simulink model "MAY31v1"  (R2023a)
settings: Solver=ode23t  StartTime=0.0  StopTime=1.6  RelTol=1e-3  AbsTol=1e-4  EnableMultiTasking=on
InitFcn:
  | Scan_Script_v8
StopFcn:
  | graphB
model workspace (MATLAB code in the model file):
  | screw_lead = 25e-3;   % m/rev
values from neighbouring files (symbols this model uses):
  mx = 1.557096    [Parameters.m]
  my = 0.574990    (= 0.57499)    [Parameters.m]
  mz = 1.557196    [Parameters.m]
  R_D = 1e-2    (= 0.01)    [Parameters.m]
  R_I = 1.2*1e-6    (= 1.2e-06)    [Parameters.m]
  Step_Rate = 200    [Parameters.m]
undefined symbols (not defined in the file or in its folder): X, xz, Y, y, Z
libraries: fl_lib x72, nesl_utility x58, sm_lib x41, fl_ps_legacy_lib x24, ee_lib x6, simulink x3, eeStairGenerator x3
(part 3 of 3)

== system MAY31v1/Stepper Motor with Control Y/Controller/Speed ==
  note: Step rate and direction algorithm implemented on a microprocessor or dedicated discrete chip
  Ref : Inport
  ERef : fl_lib/Electrical/Electrical Elements/Electrical Reference
  Step Rate and Direction : Subsystem
  Voltage-Controlled Pulse Generator : Subsystem
  PWM : PMIOPort  Side=Right
  0v : PMIOPort  Port=2  Side=Right
  REV : PMIOPort  Port=3  Side=Right
  wires:
  Ref/1 -> Step Rate and Direction/1(Reference)
  connections:
  PWM/RConn1 -- Voltage-Controlled Pulse Generator/RConn1
  Voltage-Controlled Pulse Generator/RConn2 -- 0v/RConn1 -- ERef/LConn1
  Step Rate and Direction/RConn1 -- REV/RConn1
  Step Rate and Direction/RConn2 -- Voltage-Controlled Pulse Generator/LConn1

== system MAY31v1/Stepper Motor with Control Z/Controller/Position ==
  Ref : Inport
  Algorithm and Pulse Generation : Subsystem
  ERef : fl_lib/Electrical/Electrical Elements/Electrical Reference
  PWM : PMIOPort  Side=Right
  0v : PMIOPort  Port=2  Side=Right
  REV : PMIOPort  Port=3  Side=Right
  wires:
  Ref/1 -> Algorithm and Pulse Generation/1(Reference)
  connections:
  Algorithm and Pulse Generation/RConn2 -- PWM/RConn1
  Algorithm and Pulse Generation/RConn1 -- REV/RConn1
  ERef/LConn1 -- 0v/RConn1

== system MAY31v1/Stepper Motor with Control Z/Controller/Speed ==
  note: Step rate and direction algorithm implemented on a microprocessor or dedicated discrete chip
  Ref : Inport
  ERef : fl_lib/Electrical/Electrical Elements/Electrical Reference
  Step Rate and Direction : Subsystem
  Voltage-Controlled Pulse Generator : Subsystem
  PWM : PMIOPort  Side=Right
  0v : PMIOPort  Port=2  Side=Right
  REV : PMIOPort  Port=3  Side=Right
  wires:
  Ref/1 -> Step Rate and Direction/1(Reference)
  connections:
  PWM/RConn1 -- Voltage-Controlled Pulse Generator/RConn1
  Voltage-Controlled Pulse Generator/RConn2 -- 0v/RConn1 -- ERef/LConn1
  Step Rate and Direction/RConn1 -- REV/RConn1
  Step Rate and Direction/RConn2 -- Voltage-Controlled Pulse Generator/LConn1

== system MAY31v1/X axis Lead Screw/Lead Screw Friction/Lag Filter ==
  In : Inport
  Gain : Gain  Gain=1/b
  Integrator : Integrator  InitialCondition=x_initial
  Sum : Sum  Inputs=|+-  InputSameDT=on  SaturateOnIntegerOverflow=on  OutDataTypeStr=Inherit: Same as first input
  Out : Outport  VectorParamsAs1DForOutWhenUnconnected=off
  wires:
  Sum/1 -> Integrator/1
  In/1 -> Sum/1
  Integrator/1 -> Gain/1
  Gain/1 -> Sum/2, Out/1

== system MAY31v1/X axis Lead Screw/Lead Screw Friction/Stick-Slip Friction  ==
  Fn : Inport
  v : Inport  Port=2
  Coefficient of Friction vs Velocity : Lookup_n-D  NumberOfTableDimensions=1  BreakpointsForDimension1=[-3 -1.5 -1 1 1.5 3]*vth  Table="[-muk -muk -mus mus  muk muk]"  InternalRulePriority=Speed
  Gain2 : Gain  Multiplication=Matrix(K*u)  SaturateOnIntegerOverflow=on  OutDataTypeStr=Inherit: Same as input  ParamDataTypeStr=Inherit: Same as input
  Product : Product  RndMeth=Zero
  Ff : Outport  VectorParamsAs1DForOutWhenUnconnected=off
  wires:
  Fn/1 -> Product/2  "Normal_Force"
  Coefficient of Friction vs Velocity/1 -> Product/1
  v/1 -> Coefficient of Friction vs Velocity/1  "Velocity"
  Product/1 -> Gain2/1
  Gain2/1 -> Ff/1  "Friction_Force"

== system MAY31v1/Y Axis Lead Screw/Lead Screw Friction2/Lag Filter ==
  In : Inport
  Gain : Gain  Gain=1/b
  Integrator : Integrator  InitialCondition=x_initial
  Sum : Sum  Inputs=|+-  InputSameDT=on  SaturateOnIntegerOverflow=on  OutDataTypeStr=Inherit: Same as first input
  Out : Outport  VectorParamsAs1DForOutWhenUnconnected=off
  wires:
  Sum/1 -> Integrator/1
  In/1 -> Sum/1
  Integrator/1 -> Gain/1
  Gain/1 -> Sum/2, Out/1

== system MAY31v1/Y Axis Lead Screw/Lead Screw Friction2/Stick-Slip Friction  ==
  Fn : Inport
  v : Inport  Port=2
  Coefficient of Friction vs Velocity : Lookup_n-D  NumberOfTableDimensions=1  BreakpointsForDimension1=[-3 -1.5 -1 1 1.5 3]*vth  Table="[-muk -muk -mus mus  muk muk]"  InternalRulePriority=Speed
  Gain2 : Gain  Multiplication=Matrix(K*u)  SaturateOnIntegerOverflow=on  OutDataTypeStr=Inherit: Same as input  ParamDataTypeStr=Inherit: Same as input
  Product : Product  RndMeth=Zero
  Ff : Outport  VectorParamsAs1DForOutWhenUnconnected=off
  wires:
  Fn/1 -> Product/2  "Normal_Force"
  Coefficient of Friction vs Velocity/1 -> Product/1
  v/1 -> Coefficient of Friction vs Velocity/1  "Velocity"
  Product/1 -> Gain2/1
  Gain2/1 -> Ff/1  "Friction_Force"

== system MAY31v1/Z axis Lead Screw/Lead Screw Friction1/Lag Filter ==
  In : Inport
  Gain : Gain  Gain=1/b
  Integrator : Integrator  InitialCondition=x_initial
  Sum : Sum  Inputs=|+-  InputSameDT=on  SaturateOnIntegerOverflow=on  OutDataTypeStr=Inherit: Same as first input
  Out : Outport  VectorParamsAs1DForOutWhenUnconnected=off
  wires:
  Sum/1 -> Integrator/1
  In/1 -> Sum/1
  Integrator/1 -> Gain/1
  Gain/1 -> Sum/2, Out/1

== system MAY31v1/Z axis Lead Screw/Lead Screw Friction1/Stick-Slip Friction  ==
  Fn : Inport
  v : Inport  Port=2
  Coefficient of Friction vs Velocity : Lookup_n-D  NumberOfTableDimensions=1  BreakpointsForDimension1=[-3 -1.5 -1 1 1.5 3]*vth  Table="[-muk -muk -mus mus  muk muk]"  InternalRulePriority=Speed
  Gain2 : Gain  Multiplication=Matrix(K*u)  SaturateOnIntegerOverflow=on  OutDataTypeStr=Inherit: Same as input  ParamDataTypeStr=Inherit: Same as input
  Product : Product  RndMeth=Zero
  Ff : Outport  VectorParamsAs1DForOutWhenUnconnected=off
  wires:
  Fn/1 -> Product/2  "Normal_Force"
  Coefficient of Friction vs Velocity/1 -> Product/1
  v/1 -> Coefficient of Friction vs Velocity/1  "Velocity"
  Product/1 -> Gain2/1
  Gain2/1 -> Ff/1  "Friction_Force"

== system MAY31v1/Stepper Motor with Control X/Controller/Position/Algorithm and Pulse Generation ==
  note: The reference input defines the required angular position in terms of
      | the number steps. For this stepper, the step size is 1.8 degrees. Hence
      | a demand of 10 steps results in an angle change of 18 degrees.
      | The step rate is set by the Pulse Generator's Pulse rate mask parameter.
  note: Position Controller
  Reference : Inport
  IC Analog Output REV : Subsystem
  IC Analog Output Vref : Subsystem
  Logic2Volts1 : Gain  Gain=5
  Logic2Volts2 : Gain  Gain=5
  Pulse Generator : Subsystem  mask{f=Step_Rate}
      mask prompts: f "Pulse rate"
  Rate Transition : RateTransition  Deterministic=off
  REV : PMIOPort  Side=Right
  Vref : PMIOPort  Port=2  Side=Right
  wires:
  Logic2Volts1/1 -> IC Analog Output Vref/1(SL)
  Pulse Generator/1(Pulse train) -> Logic2Volts1/1
  Reference/1 -> Rate Transition/1
  Logic2Volts2/1 -> IC Analog Output REV/1(SL)
  Pulse Generator/2(Pulse direction) -> Logic2Volts2/1
  Rate Transition/1 -> Pulse Generator/1(Pulse  demand)
  connections:
  Vref/RConn1 -- IC Analog Output Vref/RConn1
  REV/RConn1 -- IC Analog Output REV/RConn1

== system MAY31v1/Stepper Motor with Control X/Controller/Speed/Step Rate and Direction ==
  note: The speed controller turns the reference input into an absolute voltage demand for the
      | voltage-controlled pulse generator and sets the reverse flag signal to +5 volts when the
      | speed demand is negative.
  Reference : Inport
  Abs : Abs  SaturateOnIntegerOverflow=off
  Compare To Constant : simulink/Logic and Bit Operations/Compare To Constant  relop=<  const=0  OutDataTypeStr=uint8  ZeroCross=off
  Data Type Conversion : DataTypeConversion  SaturateOnIntegerOverflow=off  RndMeth=Floor
  IC Analog Output REV : Subsystem
  IC Analog Output Vref : Subsystem
  Logic2Volts : Gain  Gain=5
  Max step rate 100/s : Saturate  UpperLimit=100  LowerLimit=0
  StepRate2Volts : Gain  Gain=5/100
  REV : PMIOPort  Side=Right
  Vref : PMIOPort  Port=2  Side=Right
  wires:
  StepRate2Volts/1 -> IC Analog Output Vref/1(SL)
  Max step rate 100/s/1 -> StepRate2Volts/1
  Data Type Conversion/1 -> Logic2Volts/1
  Compare To Constant/1 -> Data Type Conversion/1
  Reference/1 -> Compare To Constant/1, Abs/1
  Abs/1 -> Max step rate 100/s/1
  Logic2Volts/1 -> IC Analog Output REV/1(SL)
  connections:
  REV/RConn1 -- IC Analog Output REV/RConn1
  Vref/RConn1 -- IC Analog Output Vref/RConn1

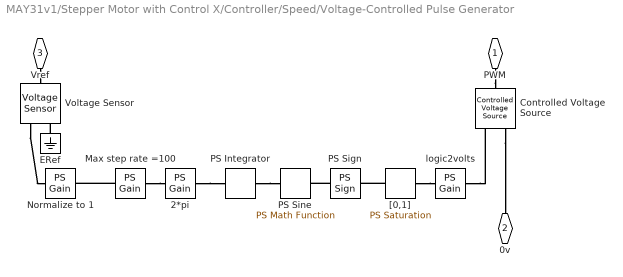
== system MAY31v1/Stepper Motor with Control X/Controller/Speed/Voltage-Controlled Pulse Generator ==
  2*pi : fl_ps_legacy_lib/Legacy Physical Signals/Functions/PS Gain  gain=-2*pi
  Controlled Voltage Source : fl_lib/Electrical/Electrical Sources/Controlled Voltage Source
  ERef : fl_lib/Electrical/Electrical Elements/Electrical Reference
  Max step rate =100 : fl_ps_legacy_lib/Legacy Physical Signals/Functions/PS Gain  gain=100
  Normalize to 1 : fl_ps_legacy_lib/Legacy Physical Signals/Functions/PS Gain  gain=1/5
  PS Integrator : fl_ps_legacy_lib/Legacy Physical Signals/Linear Operators/PS Integrator  x0=0
      settings: InternalSimscapePortConfiguration="{\"Bottom\":[],\"Left\":[{\"id\":\"I\",\"label\":\"\",\"type\":\"input\"}],\"Right\":[{\"id\":\"O\",\"label\":\"\",\"type\":\"output\"}],\"Top\":[]}"
  PS Sign : fl_ps_legacy_lib/Legacy Physical Signals/Nonlinear Operators/PS Sign
      settings: InternalSimscapePortConfiguration="{\"Bottom\":[],\"Left\":[{\"id\":\"I\",\"label\":\"\",\"type\":\"input\"}],\"Right\":[{\"id\":\"O\",\"label\":\"\",\"type\":\"output\"}],\"Top\":[]}"
  PS Sine : fl_ps_legacy_lib/Legacy Physical Signals/Functions/PS Math Function  fcn_choice=1
      settings: InternalSimscapePortConfiguration="{\"Bottom\":[],\"Left\":[{\"id\":\"I\",\"label\":\"\",\"type\":\"input\"}],\"Right\":[{\"id\":\"O\",\"label\":\"\",\"type\":\"output\"}],\"Top\":[]}"
  Voltage Sensor : fl_lib/Electrical/Electrical Sensors/Voltage Sensor
  "[0,1]" : fl_ps_legacy_lib/Legacy Physical Signals/Nonlinear Operators/PS Saturation  upper_limit=1  lower_limit=0
      settings: InternalSimscapePortConfiguration="{\"Bottom\":[],\"Left\":[{\"id\":\"I\",\"label\":\"\",\"type\":\"input\"}],\"Right\":[{\"id\":\"O\",\"label\":\"\",\"type\":\"output\"}],\"Top\":[]}"
  logic2volts : fl_ps_legacy_lib/Legacy Physical Signals/Functions/PS Gain  gain=5
  PWM : PMIOPort  Side=Right
  0v : PMIOPort  Port=2  Side=Right
  Vref : PMIOPort  Port=3  Side=Left
  connections:
  PWM/RConn1 -- Controlled Voltage Source/LConn1
  Controlled Voltage Source/RConn2 -- 0v/RConn1
  Vref/RConn1 -- Voltage Sensor/LConn1
  ERef/LConn1 -- Voltage Sensor/RConn2
  Voltage Sensor/RConn1 -- Normalize to 1/LConn1
  Max step rate =100/LConn1 -- Normalize to 1/RConn1
  Max step rate =100/RConn1 -- 2*pi/LConn1
  2*pi/RConn1 -- PS Integrator/LConn1
  PS Integrator/RConn1 -- PS Sine/LConn1
  PS Sign/LConn1 -- PS Sine/RConn1
  "[0,1]"/LConn1 -- PS Sign/RConn1
  "[0,1]"/RConn1 -- logic2volts/LConn1
  logic2volts/RConn1 -- Controlled Voltage Source/RConn1

== system MAY31v1/Stepper Motor with Control Y/Controller/Position/Algorithm and Pulse Generation ==
  note: The reference input defines the required angular position in terms of
      | the number steps. For this stepper, the step size is 1.8 degrees. Hence
      | a demand of 10 steps results in an angle change of 18 degrees.
      | The step rate is set by the Pulse Generator's Pulse rate mask parameter.
  note: Position Controller
  Reference : Inport
  IC Analog Output REV : Subsystem
  IC Analog Output Vref : Subsystem
  Logic2Volts1 : Gain  Gain=5
  Logic2Volts2 : Gain  Gain=5
  Pulse Generator : Subsystem  mask{f=Step_Rate}
      mask prompts: f "Pulse rate"
  Rate Transition : RateTransition  Deterministic=off
  REV : PMIOPort  Side=Right
  Vref : PMIOPort  Port=2  Side=Right
  wires:
  Logic2Volts1/1 -> IC Analog Output Vref/1(SL)
  Pulse Generator/1(Pulse train) -> Logic2Volts1/1
  Reference/1 -> Rate Transition/1
  Logic2Volts2/1 -> IC Analog Output REV/1(SL)
  Pulse Generator/2(Pulse direction) -> Logic2Volts2/1
  Rate Transition/1 -> Pulse Generator/1(Pulse  demand)
  connections:
  Vref/RConn1 -- IC Analog Output Vref/RConn1
  REV/RConn1 -- IC Analog Output REV/RConn1

== system MAY31v1/Stepper Motor with Control Y/Controller/Speed/Step Rate and Direction ==
  note: The speed controller turns the reference input into an absolute voltage demand for the
      | voltage-controlled pulse generator and sets the reverse flag signal to +5 volts when the
      | speed demand is negative.
  Reference : Inport
  Abs : Abs  SaturateOnIntegerOverflow=off
  Compare To Constant : simulink/Logic and Bit Operations/Compare To Constant  relop=<  const=0  OutDataTypeStr=uint8  ZeroCross=off
  Data Type Conversion : DataTypeConversion  SaturateOnIntegerOverflow=off  RndMeth=Floor
  IC Analog Output REV : Subsystem
  IC Analog Output Vref : Subsystem
  Logic2Volts : Gain  Gain=5
  Max step rate 100/s : Saturate  UpperLimit=100  LowerLimit=0
  StepRate2Volts : Gain  Gain=5/100
  REV : PMIOPort  Side=Right
  Vref : PMIOPort  Port=2  Side=Right
  wires:
  StepRate2Volts/1 -> IC Analog Output Vref/1(SL)
  Max step rate 100/s/1 -> StepRate2Volts/1
  Data Type Conversion/1 -> Logic2Volts/1
  Compare To Constant/1 -> Data Type Conversion/1
  Reference/1 -> Compare To Constant/1, Abs/1
  Abs/1 -> Max step rate 100/s/1
  Logic2Volts/1 -> IC Analog Output REV/1(SL)
  connections:
  REV/RConn1 -- IC Analog Output REV/RConn1
  Vref/RConn1 -- IC Analog Output Vref/RConn1

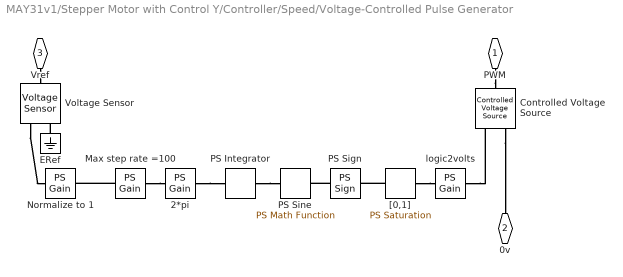
== system MAY31v1/Stepper Motor with Control Y/Controller/Speed/Voltage-Controlled Pulse Generator ==
  2*pi : fl_ps_legacy_lib/Legacy Physical Signals/Functions/PS Gain  gain=-2*pi
  Controlled Voltage Source : fl_lib/Electrical/Electrical Sources/Controlled Voltage Source
  ERef : fl_lib/Electrical/Electrical Elements/Electrical Reference
  Max step rate =100 : fl_ps_legacy_lib/Legacy Physical Signals/Functions/PS Gain  gain=100
  Normalize to 1 : fl_ps_legacy_lib/Legacy Physical Signals/Functions/PS Gain  gain=1/5
  PS Integrator : fl_ps_legacy_lib/Legacy Physical Signals/Linear Operators/PS Integrator  x0=0
      settings: InternalSimscapePortConfiguration="{\"Bottom\":[],\"Left\":[{\"id\":\"I\",\"label\":\"\",\"type\":\"input\"}],\"Right\":[{\"id\":\"O\",\"label\":\"\",\"type\":\"output\"}],\"Top\":[]}"
  PS Sign : fl_ps_legacy_lib/Legacy Physical Signals/Nonlinear Operators/PS Sign
      settings: InternalSimscapePortConfiguration="{\"Bottom\":[],\"Left\":[{\"id\":\"I\",\"label\":\"\",\"type\":\"input\"}],\"Right\":[{\"id\":\"O\",\"label\":\"\",\"type\":\"output\"}],\"Top\":[]}"
  PS Sine : fl_ps_legacy_lib/Legacy Physical Signals/Functions/PS Math Function  fcn_choice=1
      settings: InternalSimscapePortConfiguration="{\"Bottom\":[],\"Left\":[{\"id\":\"I\",\"label\":\"\",\"type\":\"input\"}],\"Right\":[{\"id\":\"O\",\"label\":\"\",\"type\":\"output\"}],\"Top\":[]}"
  Voltage Sensor : fl_lib/Electrical/Electrical Sensors/Voltage Sensor
  "[0,1]" : fl_ps_legacy_lib/Legacy Physical Signals/Nonlinear Operators/PS Saturation  upper_limit=1  lower_limit=0
      settings: InternalSimscapePortConfiguration="{\"Bottom\":[],\"Left\":[{\"id\":\"I\",\"label\":\"\",\"type\":\"input\"}],\"Right\":[{\"id\":\"O\",\"label\":\"\",\"type\":\"output\"}],\"Top\":[]}"
  logic2volts : fl_ps_legacy_lib/Legacy Physical Signals/Functions/PS Gain  gain=5
  PWM : PMIOPort  Side=Right
  0v : PMIOPort  Port=2  Side=Right
  Vref : PMIOPort  Port=3  Side=Left
  connections:
  PWM/RConn1 -- Controlled Voltage Source/LConn1
  Controlled Voltage Source/RConn2 -- 0v/RConn1
  Vref/RConn1 -- Voltage Sensor/LConn1
  ERef/LConn1 -- Voltage Sensor/RConn2
  Voltage Sensor/RConn1 -- Normalize to 1/LConn1
  Max step rate =100/LConn1 -- Normalize to 1/RConn1
  Max step rate =100/RConn1 -- 2*pi/LConn1
  2*pi/RConn1 -- PS Integrator/LConn1
  PS Integrator/RConn1 -- PS Sine/LConn1
  PS Sign/LConn1 -- PS Sine/RConn1
  "[0,1]"/LConn1 -- PS Sign/RConn1
  "[0,1]"/RConn1 -- logic2volts/LConn1
  logic2volts/RConn1 -- Controlled Voltage Source/RConn1

== system MAY31v1/Stepper Motor with Control Z/Controller/Position/Algorithm and Pulse Generation ==
  note: The reference input defines the required angular position in terms of
      | the number steps. For this stepper, the step size is 1.8 degrees. Hence
      | a demand of 10 steps results in an angle change of 18 degrees.
      | The step rate is set by the Pulse Generator's Pulse rate mask parameter.
  note: Position Controller
  Reference : Inport
  IC Analog Output REV : Subsystem
  IC Analog Output Vref : Subsystem
  Logic2Volts1 : Gain  Gain=5
  Logic2Volts2 : Gain  Gain=5
  Pulse Generator : Subsystem  mask{f=Step_Rate}
      mask prompts: f "Pulse rate"
  Rate Transition : RateTransition  Deterministic=off
  REV : PMIOPort  Side=Right
  Vref : PMIOPort  Port=2  Side=Right
  wires:
  Logic2Volts1/1 -> IC Analog Output Vref/1(SL)
  Pulse Generator/1(Pulse train) -> Logic2Volts1/1
  Reference/1 -> Rate Transition/1
  Logic2Volts2/1 -> IC Analog Output REV/1(SL)
  Pulse Generator/2(Pulse direction) -> Logic2Volts2/1
  Rate Transition/1 -> Pulse Generator/1(Pulse  demand)
  connections:
  Vref/RConn1 -- IC Analog Output Vref/RConn1
  REV/RConn1 -- IC Analog Output REV/RConn1

== system MAY31v1/Stepper Motor with Control Z/Controller/Speed/Step Rate and Direction ==
  note: The speed controller turns the reference input into an absolute voltage demand for the
      | voltage-controlled pulse generator and sets the reverse flag signal to +5 volts when the
      | speed demand is negative.
  Reference : Inport
  Abs : Abs  SaturateOnIntegerOverflow=off
  Compare To Constant : simulink/Logic and Bit Operations/Compare To Constant  relop=<  const=0  OutDataTypeStr=uint8  ZeroCross=off
  Data Type Conversion : DataTypeConversion  SaturateOnIntegerOverflow=off  RndMeth=Floor
  IC Analog Output REV : Subsystem
  IC Analog Output Vref : Subsystem
  Logic2Volts : Gain  Gain=5
  Max step rate 100/s : Saturate  UpperLimit=100  LowerLimit=0
  StepRate2Volts : Gain  Gain=5/100
  REV : PMIOPort  Side=Right
  Vref : PMIOPort  Port=2  Side=Right
  wires:
  StepRate2Volts/1 -> IC Analog Output Vref/1(SL)
  Max step rate 100/s/1 -> StepRate2Volts/1
  Data Type Conversion/1 -> Logic2Volts/1
  Compare To Constant/1 -> Data Type Conversion/1
  Reference/1 -> Compare To Constant/1, Abs/1
  Abs/1 -> Max step rate 100/s/1
  Logic2Volts/1 -> IC Analog Output REV/1(SL)
  connections:
  REV/RConn1 -- IC Analog Output REV/RConn1
  Vref/RConn1 -- IC Analog Output Vref/RConn1

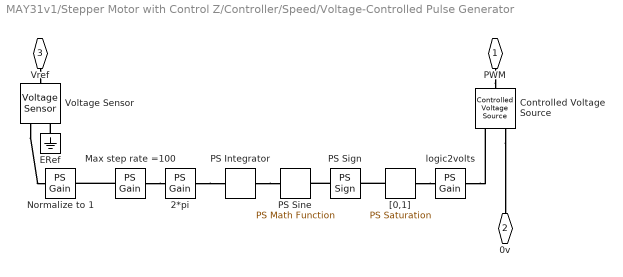
== system MAY31v1/Stepper Motor with Control Z/Controller/Speed/Voltage-Controlled Pulse Generator ==
  2*pi : fl_ps_legacy_lib/Legacy Physical Signals/Functions/PS Gain  gain=-2*pi
  Controlled Voltage Source : fl_lib/Electrical/Electrical Sources/Controlled Voltage Source
  ERef : fl_lib/Electrical/Electrical Elements/Electrical Reference
  Max step rate =100 : fl_ps_legacy_lib/Legacy Physical Signals/Functions/PS Gain  gain=100
  Normalize to 1 : fl_ps_legacy_lib/Legacy Physical Signals/Functions/PS Gain  gain=1/5
  PS Integrator : fl_ps_legacy_lib/Legacy Physical Signals/Linear Operators/PS Integrator  x0=0
      settings: InternalSimscapePortConfiguration="{\"Bottom\":[],\"Left\":[{\"id\":\"I\",\"label\":\"\",\"type\":\"input\"}],\"Right\":[{\"id\":\"O\",\"label\":\"\",\"type\":\"output\"}],\"Top\":[]}"
  PS Sign : fl_ps_legacy_lib/Legacy Physical Signals/Nonlinear Operators/PS Sign
      settings: InternalSimscapePortConfiguration="{\"Bottom\":[],\"Left\":[{\"id\":\"I\",\"label\":\"\",\"type\":\"input\"}],\"Right\":[{\"id\":\"O\",\"label\":\"\",\"type\":\"output\"}],\"Top\":[]}"
  PS Sine : fl_ps_legacy_lib/Legacy Physical Signals/Functions/PS Math Function  fcn_choice=1
      settings: InternalSimscapePortConfiguration="{\"Bottom\":[],\"Left\":[{\"id\":\"I\",\"label\":\"\",\"type\":\"input\"}],\"Right\":[{\"id\":\"O\",\"label\":\"\",\"type\":\"output\"}],\"Top\":[]}"
  Voltage Sensor : fl_lib/Electrical/Electrical Sensors/Voltage Sensor
  "[0,1]" : fl_ps_legacy_lib/Legacy Physical Signals/Nonlinear Operators/PS Saturation  upper_limit=1  lower_limit=0
      settings: InternalSimscapePortConfiguration="{\"Bottom\":[],\"Left\":[{\"id\":\"I\",\"label\":\"\",\"type\":\"input\"}],\"Right\":[{\"id\":\"O\",\"label\":\"\",\"type\":\"output\"}],\"Top\":[]}"
  logic2volts : fl_ps_legacy_lib/Legacy Physical Signals/Functions/PS Gain  gain=5
  PWM : PMIOPort  Side=Right
  0v : PMIOPort  Port=2  Side=Right
  Vref : PMIOPort  Port=3  Side=Left
  connections:
  PWM/RConn1 -- Controlled Voltage Source/LConn1
  Controlled Voltage Source/RConn2 -- 0v/RConn1
  Vref/RConn1 -- Voltage Sensor/LConn1
  ERef/LConn1 -- Voltage Sensor/RConn2
  Voltage Sensor/RConn1 -- Normalize to 1/LConn1
  Max step rate =100/LConn1 -- Normalize to 1/RConn1
  Max step rate =100/RConn1 -- 2*pi/LConn1
  2*pi/RConn1 -- PS Integrator/LConn1
  PS Integrator/RConn1 -- PS Sine/LConn1
  PS Sign/LConn1 -- PS Sine/RConn1
  "[0,1]"/LConn1 -- PS Sign/RConn1
  "[0,1]"/RConn1 -- logic2volts/LConn1
  logic2volts/RConn1 -- Controlled Voltage Source/RConn1

== system MAY31v1/Stepper Motor with Control X/Controller/Position/Algorithm and Pulse Generation/IC Analog Output REV ==
  SL : Inport
  Controlled Voltage Source : fl_lib/Electrical/Electrical Sources/Controlled Voltage Source
  ERef : fl_lib/Electrical/Electrical Elements/Electrical Reference
  Simulink-PS Converter : nesl_utility/Simulink-PS Converter  PhysicalDomain=network_engine_domain  SubClassName=ps_input  LeftPortType=input  RightPortType=output  PseudoPeriodic=off  Frequencies=[]  NoiseDistribution=none  NoiseParameters=[]  Unit=V  AffineConversion=off  FilteringAndDerivatives=zero  SimscapeFilterOrder=1  InputFilterTimeConstant=.001  UdotUserProvided=0
  V : PMIOPort  Side=Right
  wires:
  SL/1 -> Simulink-PS Converter/1
  connections:
  ERef/LConn1 -- Controlled Voltage Source/RConn2
  V/RConn1 -- Controlled Voltage Source/LConn1
  Simulink-PS Converter/RConn1 -- Controlled Voltage Source/RConn1

== system MAY31v1/Stepper Motor with Control X/Controller/Position/Algorithm and Pulse Generation/IC Analog Output Vref ==
  SL : Inport
  Controlled Voltage Source : fl_lib/Electrical/Electrical Sources/Controlled Voltage Source
  ERef : fl_lib/Electrical/Electrical Elements/Electrical Reference
  Simulink-PS Converter : nesl_utility/Simulink-PS Converter  PhysicalDomain=network_engine_domain  SubClassName=ps_input  LeftPortType=input  RightPortType=output  PseudoPeriodic=off  Frequencies=[]  NoiseDistribution=none  NoiseParameters=[]  Unit=V  AffineConversion=off  FilteringAndDerivatives=zero  SimscapeFilterOrder=1  InputFilterTimeConstant=.001  UdotUserProvided=0
  V : PMIOPort  Side=Right
  wires:
  SL/1 -> Simulink-PS Converter/1
  connections:
  Simulink-PS Converter/RConn1 -- Controlled Voltage Source/RConn1
  V/RConn1 -- Controlled Voltage Source/LConn1
  ERef/LConn1 -- Controlled Voltage Source/RConn2

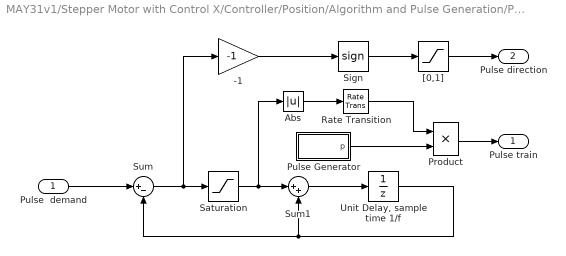
== system MAY31v1/Stepper Motor with Control X/Controller/Position/Algorithm and Pulse Generation/Pulse Generator ==
  Pulse  demand : Inport  SampleTime=1/f
  -1 : Gain  Gain=-1
  Abs : Abs  SaturateOnIntegerOverflow=off
  Product : Product  InputSameDT=on  SaturateOnIntegerOverflow=on  OutDataTypeStr=Inherit: Same as first input
  Pulse Generator : Subsystem
  Rate Transition : RateTransition  Deterministic=off
  Saturation : Saturate  UpperLimit=1  LowerLimit=-1
  Sign : Signum
  Sum : Sum  Inputs=|+-
  Sum1 : Sum  Inputs=|++
  "Unit Delay, sample time 1/f" : UnitDelay  SampleTime=1/f  HasFrameUpgradeWarning=on
  "[0,1]" : Saturate  UpperLimit=1  LowerLimit=0
  Pulse train : Outport  VectorParamsAs1DForOutWhenUnconnected=off
  Pulse direction : Outport  Port=2  VectorParamsAs1DForOutWhenUnconnected=off
  wires:
  "[0,1]"/1 -> Pulse direction/1
  -1/1 -> Sign/1
  "Unit Delay, sample time 1/f"/1 -> Sum/2, Sum1/2
  Pulse  demand/1 -> Sum/1
  Sum/1 -> -1/1, Saturation/1
  Saturation/1 -> Sum1/1, Abs/1
  Sum1/1 -> "Unit Delay, sample time 1/f"/1
  Sign/1 -> "[0,1]"/1
  Product/1 -> Pulse train/1
  Abs/1 -> Rate Transition/1
  Pulse Generator/1(p) -> Product/2
  Rate Transition/1 -> Product/1

== system MAY31v1/Stepper Motor with Control X/Controller/Speed/Step Rate and Direction/IC Analog Output REV ==
  SL : Inport
  Controlled Voltage Source : fl_lib/Electrical/Electrical Sources/Controlled Voltage Source
  ERef : fl_lib/Electrical/Electrical Elements/Electrical Reference
  Simulink-PS Converter : nesl_utility/Simulink-PS Converter  PhysicalDomain=network_engine_domain  SubClassName=ps_input  LeftPortType=input  RightPortType=output  PseudoPeriodic=off  Frequencies=[]  NoiseDistribution=none  NoiseParameters=[]  Unit=V  AffineConversion=off  FilteringAndDerivatives=zero  SimscapeFilterOrder=1  InputFilterTimeConstant=.001  UdotUserProvided=0
  V : PMIOPort  Side=Right
  wires:
  SL/1 -> Simulink-PS Converter/1
  connections:
  Simulink-PS Converter/RConn1 -- Controlled Voltage Source/RConn1
  V/RConn1 -- Controlled Voltage Source/LConn1
  ERef/LConn1 -- Controlled Voltage Source/RConn2

== system MAY31v1/Stepper Motor with Control X/Controller/Speed/Step Rate and Direction/IC Analog Output Vref ==
  SL : Inport
  Controlled Voltage Source : fl_lib/Electrical/Electrical Sources/Controlled Voltage Source
  ERef : fl_lib/Electrical/Electrical Elements/Electrical Reference
  Simulink-PS Converter : nesl_utility/Simulink-PS Converter  PhysicalDomain=network_engine_domain  SubClassName=ps_input  LeftPortType=input  RightPortType=output  PseudoPeriodic=off  Frequencies=[]  NoiseDistribution=none  NoiseParameters=[]  Unit=V  AffineConversion=off  FilteringAndDerivatives=zero  SimscapeFilterOrder=1  InputFilterTimeConstant=.001  UdotUserProvided=0
  V : PMIOPort  Side=Right
  wires:
  SL/1 -> Simulink-PS Converter/1
  connections:
  ERef/LConn1 -- Controlled Voltage Source/RConn2
  V/RConn1 -- Controlled Voltage Source/LConn1
  Simulink-PS Converter/RConn1 -- Controlled Voltage Source/RConn1

== system MAY31v1/Stepper Motor with Control Y/Controller/Position/Algorithm and Pulse Generation/IC Analog Output REV ==
  SL : Inport
  Controlled Voltage Source : fl_lib/Electrical/Electrical Sources/Controlled Voltage Source
  ERef : fl_lib/Electrical/Electrical Elements/Electrical Reference
  Simulink-PS Converter : nesl_utility/Simulink-PS Converter  PhysicalDomain=network_engine_domain  SubClassName=ps_input  LeftPortType=input  RightPortType=output  PseudoPeriodic=off  Frequencies=[]  NoiseDistribution=none  NoiseParameters=[]  Unit=V  AffineConversion=off  FilteringAndDerivatives=zero  SimscapeFilterOrder=1  InputFilterTimeConstant=.001  UdotUserProvided=0
  V : PMIOPort  Side=Right
  wires:
  SL/1 -> Simulink-PS Converter/1
  connections:
  ERef/LConn1 -- Controlled Voltage Source/RConn2
  V/RConn1 -- Controlled Voltage Source/LConn1
  Simulink-PS Converter/RConn1 -- Controlled Voltage Source/RConn1

== system MAY31v1/Stepper Motor with Control Y/Controller/Position/Algorithm and Pulse Generation/IC Analog Output Vref ==
  SL : Inport
  Controlled Voltage Source : fl_lib/Electrical/Electrical Sources/Controlled Voltage Source
  ERef : fl_lib/Electrical/Electrical Elements/Electrical Reference
  Simulink-PS Converter : nesl_utility/Simulink-PS Converter  PhysicalDomain=network_engine_domain  SubClassName=ps_input  LeftPortType=input  RightPortType=output  PseudoPeriodic=off  Frequencies=[]  NoiseDistribution=none  NoiseParameters=[]  Unit=V  AffineConversion=off  FilteringAndDerivatives=zero  SimscapeFilterOrder=1  InputFilterTimeConstant=.001  UdotUserProvided=0
  V : PMIOPort  Side=Right
  wires:
  SL/1 -> Simulink-PS Converter/1
  connections:
  Simulink-PS Converter/RConn1 -- Controlled Voltage Source/RConn1
  V/RConn1 -- Controlled Voltage Source/LConn1
  ERef/LConn1 -- Controlled Voltage Source/RConn2

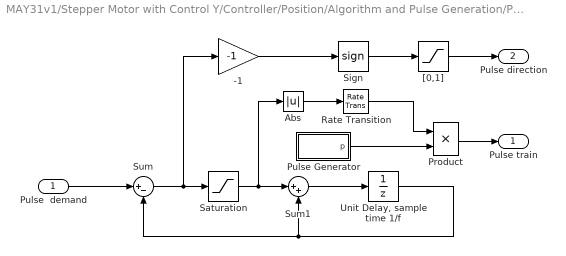
== system MAY31v1/Stepper Motor with Control Y/Controller/Position/Algorithm and Pulse Generation/Pulse Generator ==
  Pulse  demand : Inport  SampleTime=1/f
  -1 : Gain  Gain=-1
  Abs : Abs  SaturateOnIntegerOverflow=off
  Product : Product  InputSameDT=on  SaturateOnIntegerOverflow=on  OutDataTypeStr=Inherit: Same as first input
  Pulse Generator : Subsystem
  Rate Transition : RateTransition  Deterministic=off
  Saturation : Saturate  UpperLimit=1  LowerLimit=-1
  Sign : Signum
  Sum : Sum  Inputs=|+-
  Sum1 : Sum  Inputs=|++
  "Unit Delay, sample time 1/f" : UnitDelay  SampleTime=1/f  HasFrameUpgradeWarning=on
  "[0,1]" : Saturate  UpperLimit=1  LowerLimit=0
  Pulse train : Outport  VectorParamsAs1DForOutWhenUnconnected=off
  Pulse direction : Outport  Port=2  VectorParamsAs1DForOutWhenUnconnected=off
  wires:
  "[0,1]"/1 -> Pulse direction/1
  -1/1 -> Sign/1
  "Unit Delay, sample time 1/f"/1 -> Sum/2, Sum1/2
  Pulse  demand/1 -> Sum/1
  Sum/1 -> -1/1, Saturation/1
  Saturation/1 -> Sum1/1, Abs/1
  Sum1/1 -> "Unit Delay, sample time 1/f"/1
  Sign/1 -> "[0,1]"/1
  Product/1 -> Pulse train/1
  Abs/1 -> Rate Transition/1
  Pulse Generator/1(p) -> Product/2
  Rate Transition/1 -> Product/1

== system MAY31v1/Stepper Motor with Control Y/Controller/Speed/Step Rate and Direction/IC Analog Output REV ==
  SL : Inport
  Controlled Voltage Source : fl_lib/Electrical/Electrical Sources/Controlled Voltage Source
  ERef : fl_lib/Electrical/Electrical Elements/Electrical Reference
  Simulink-PS Converter : nesl_utility/Simulink-PS Converter  PhysicalDomain=network_engine_domain  SubClassName=ps_input  LeftPortType=input  RightPortType=output  PseudoPeriodic=off  Frequencies=[]  NoiseDistribution=none  NoiseParameters=[]  Unit=V  AffineConversion=off  FilteringAndDerivatives=zero  SimscapeFilterOrder=1  InputFilterTimeConstant=.001  UdotUserProvided=0
  V : PMIOPort  Side=Right
  wires:
  SL/1 -> Simulink-PS Converter/1
  connections:
  Simulink-PS Converter/RConn1 -- Controlled Voltage Source/RConn1
  V/RConn1 -- Controlled Voltage Source/LConn1
  ERef/LConn1 -- Controlled Voltage Source/RConn2

== system MAY31v1/Stepper Motor with Control Y/Controller/Speed/Step Rate and Direction/IC Analog Output Vref ==
  SL : Inport
  Controlled Voltage Source : fl_lib/Electrical/Electrical Sources/Controlled Voltage Source
  ERef : fl_lib/Electrical/Electrical Elements/Electrical Reference
  Simulink-PS Converter : nesl_utility/Simulink-PS Converter  PhysicalDomain=network_engine_domain  SubClassName=ps_input  LeftPortType=input  RightPortType=output  PseudoPeriodic=off  Frequencies=[]  NoiseDistribution=none  NoiseParameters=[]  Unit=V  AffineConversion=off  FilteringAndDerivatives=zero  SimscapeFilterOrder=1  InputFilterTimeConstant=.001  UdotUserProvided=0
  V : PMIOPort  Side=Right
  wires:
  SL/1 -> Simulink-PS Converter/1
  connections:
  ERef/LConn1 -- Controlled Voltage Source/RConn2
  V/RConn1 -- Controlled Voltage Source/LConn1
  Simulink-PS Converter/RConn1 -- Controlled Voltage Source/RConn1

== system MAY31v1/Stepper Motor with Control Z/Controller/Position/Algorithm and Pulse Generation/IC Analog Output REV ==
  SL : Inport
  Controlled Voltage Source : fl_lib/Electrical/Electrical Sources/Controlled Voltage Source
  ERef : fl_lib/Electrical/Electrical Elements/Electrical Reference
  Simulink-PS Converter : nesl_utility/Simulink-PS Converter  PhysicalDomain=network_engine_domain  SubClassName=ps_input  LeftPortType=input  RightPortType=output  PseudoPeriodic=off  Frequencies=[]  NoiseDistribution=none  NoiseParameters=[]  Unit=V  AffineConversion=off  FilteringAndDerivatives=zero  SimscapeFilterOrder=1  InputFilterTimeConstant=.001  UdotUserProvided=0
  V : PMIOPort  Side=Right
  wires:
  SL/1 -> Simulink-PS Converter/1
  connections:
  ERef/LConn1 -- Controlled Voltage Source/RConn2
  V/RConn1 -- Controlled Voltage Source/LConn1
  Simulink-PS Converter/RConn1 -- Controlled Voltage Source/RConn1

== system MAY31v1/Stepper Motor with Control Z/Controller/Position/Algorithm and Pulse Generation/IC Analog Output Vref ==
  SL : Inport
  Controlled Voltage Source : fl_lib/Electrical/Electrical Sources/Controlled Voltage Source
  ERef : fl_lib/Electrical/Electrical Elements/Electrical Reference
  Simulink-PS Converter : nesl_utility/Simulink-PS Converter  PhysicalDomain=network_engine_domain  SubClassName=ps_input  LeftPortType=input  RightPortType=output  PseudoPeriodic=off  Frequencies=[]  NoiseDistribution=none  NoiseParameters=[]  Unit=V  AffineConversion=off  FilteringAndDerivatives=zero  SimscapeFilterOrder=1  InputFilterTimeConstant=.001  UdotUserProvided=0
  V : PMIOPort  Side=Right
  wires:
  SL/1 -> Simulink-PS Converter/1
  connections:
  Simulink-PS Converter/RConn1 -- Controlled Voltage Source/RConn1
  V/RConn1 -- Controlled Voltage Source/LConn1
  ERef/LConn1 -- Controlled Voltage Source/RConn2

== system MAY31v1/Stepper Motor with Control Z/Controller/Position/Algorithm and Pulse Generation/Pulse Generator ==
  Pulse  demand : Inport  SampleTime=1/f
  -1 : Gain  Gain=-1
  Abs : Abs  SaturateOnIntegerOverflow=off
  Product : Product  InputSameDT=on  SaturateOnIntegerOverflow=on  OutDataTypeStr=Inherit: Same as first input
  Pulse Generator : Subsystem
  Rate Transition : RateTransition  Deterministic=off
  Saturation : Saturate  UpperLimit=1  LowerLimit=-1
  Sign : Signum
  Sum : Sum  Inputs=|+-
  Sum1 : Sum  Inputs=|++
  "Unit Delay, sample time 1/f" : UnitDelay  SampleTime=1/f  HasFrameUpgradeWarning=on
  "[0,1]" : Saturate  UpperLimit=1  LowerLimit=0
  Pulse train : Outport  VectorParamsAs1DForOutWhenUnconnected=off
  Pulse direction : Outport  Port=2  VectorParamsAs1DForOutWhenUnconnected=off
  wires:
  "[0,1]"/1 -> Pulse direction/1
  -1/1 -> Sign/1
  "Unit Delay, sample time 1/f"/1 -> Sum/2, Sum1/2
  Pulse  demand/1 -> Sum/1
  Sum/1 -> -1/1, Saturation/1
  Saturation/1 -> Sum1/1, Abs/1
  Sum1/1 -> "Unit Delay, sample time 1/f"/1
  Sign/1 -> "[0,1]"/1
  Product/1 -> Pulse train/1
  Abs/1 -> Rate Transition/1
  Pulse Generator/1(p) -> Product/2
  Rate Transition/1 -> Product/1

== system MAY31v1/Stepper Motor with Control Z/Controller/Speed/Step Rate and Direction/IC Analog Output REV ==
  SL : Inport
  Controlled Voltage Source : fl_lib/Electrical/Electrical Sources/Controlled Voltage Source
  ERef : fl_lib/Electrical/Electrical Elements/Electrical Reference
  Simulink-PS Converter : nesl_utility/Simulink-PS Converter  PhysicalDomain=network_engine_domain  SubClassName=ps_input  LeftPortType=input  RightPortType=output  PseudoPeriodic=off  Frequencies=[]  NoiseDistribution=none  NoiseParameters=[]  Unit=V  AffineConversion=off  FilteringAndDerivatives=zero  SimscapeFilterOrder=1  InputFilterTimeConstant=.001  UdotUserProvided=0
  V : PMIOPort  Side=Right
  wires:
  SL/1 -> Simulink-PS Converter/1
  connections:
  Simulink-PS Converter/RConn1 -- Controlled Voltage Source/RConn1
  V/RConn1 -- Controlled Voltage Source/LConn1
  ERef/LConn1 -- Controlled Voltage Source/RConn2

== system MAY31v1/Stepper Motor with Control Z/Controller/Speed/Step Rate and Direction/IC Analog Output Vref ==
  SL : Inport
  Controlled Voltage Source : fl_lib/Electrical/Electrical Sources/Controlled Voltage Source
  ERef : fl_lib/Electrical/Electrical Elements/Electrical Reference
  Simulink-PS Converter : nesl_utility/Simulink-PS Converter  PhysicalDomain=network_engine_domain  SubClassName=ps_input  LeftPortType=input  RightPortType=output  PseudoPeriodic=off  Frequencies=[]  NoiseDistribution=none  NoiseParameters=[]  Unit=V  AffineConversion=off  FilteringAndDerivatives=zero  SimscapeFilterOrder=1  InputFilterTimeConstant=.001  UdotUserProvided=0
  V : PMIOPort  Side=Right
  wires:
  SL/1 -> Simulink-PS Converter/1
  connections:
  ERef/LConn1 -- Controlled Voltage Source/RConn2
  V/RConn1 -- Controlled Voltage Source/LConn1
  Simulink-PS Converter/RConn1 -- Controlled Voltage Source/RConn1

== system MAY31v1/Stepper Motor with Control X/Controller/Position/Algorithm and Pulse Generation/Pulse Generator/Pulse Generator ==
  -1 : Gain  Gain=0.5
  Constant : Constant  SampleTime=1/(2*f)
  Gain : Gain  Gain=-1
  Sum : Sum  Inputs=|++
  "Unit Delay, sample time 1/2*f)" : UnitDelay  InitialCondition=-1  SampleTime=1/(2*f)  HasFrameUpgradeWarning=on
  p : Outport  VectorParamsAs1DForOutWhenUnconnected=off
  wires:
  "Unit Delay, sample time 1/2*f)"/1 -> Gain/1, Sum/1
  Gain/1 -> "Unit Delay, sample time 1/2*f)"/1
  Constant/1 -> Sum/2
  Sum/1 -> -1/1
  -1/1 -> p/1

== system MAY31v1/Stepper Motor with Control Y/Controller/Position/Algorithm and Pulse Generation/Pulse Generator/Pulse Generator ==
  -1 : Gain  Gain=0.5
  Constant : Constant  SampleTime=1/(2*f)
  Gain : Gain  Gain=-1
  Sum : Sum  Inputs=|++
  "Unit Delay, sample time 1/2*f)" : UnitDelay  InitialCondition=-1  SampleTime=1/(2*f)  HasFrameUpgradeWarning=on
  p : Outport  VectorParamsAs1DForOutWhenUnconnected=off
  wires:
  "Unit Delay, sample time 1/2*f)"/1 -> Gain/1, Sum/1
  Gain/1 -> "Unit Delay, sample time 1/2*f)"/1
  Constant/1 -> Sum/2
  Sum/1 -> -1/1
  -1/1 -> p/1

== system MAY31v1/Stepper Motor with Control Z/Controller/Position/Algorithm and Pulse Generation/Pulse Generator/Pulse Generator ==
  -1 : Gain  Gain=0.5
  Constant : Constant  SampleTime=1/(2*f)
  Gain : Gain  Gain=-1
  Sum : Sum  Inputs=|++
  "Unit Delay, sample time 1/2*f)" : UnitDelay  InitialCondition=-1  SampleTime=1/(2*f)  HasFrameUpgradeWarning=on
  p : Outport  VectorParamsAs1DForOutWhenUnconnected=off
  wires:
  "Unit Delay, sample time 1/2*f)"/1 -> Gain/1, Sum/1
  Gain/1 -> "Unit Delay, sample time 1/2*f)"/1
  Constant/1 -> Sum/2
  Sum/1 -> -1/1
  -1/1 -> p/1
